simulink model "KalmanPoging1"  (R2019b)
settings: Solver=VariableStepAuto  StartTime=0.0  StopTime=6031  RelTol=1e-3
libraries: simulink x1
settings Model: Creator=pieterpinson  LastModifiedBy=pieterpinson

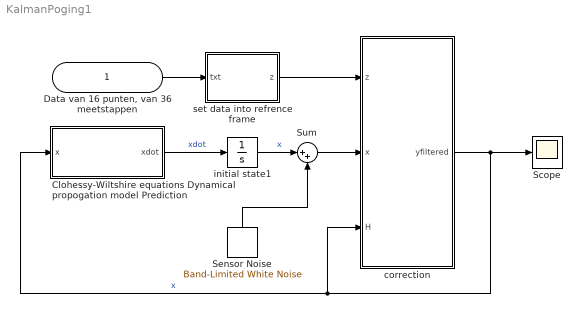
== system KalmanPoging1 ==
  "Data van 16 punten, van 36 meetstappen" : Inport
  Clohessy-Wiltshire equations Dynamical propogation model Prediction : MATLAB Function  TreatAsAtomicUnit=on
  Scope : Scope
  Sensor Noise : simulink/Sources/Band-Limited White Noise  Cov=[0.1]  Ts=0.1  seed=[23341]
  Sum : Sum  Inputs=|++
  correction : MATLAB Function  TreatAsAtomicUnit=on
  initial state1 : Integrator  InitialCondition=|
      | [-2.9671 ; 0.5236
      | ; -1.3963 ; -0.0873 ; -0.1489 ; 0.0262]
  set data into refrence frame : MATLAB Function  TreatAsAtomicUnit=on
  wires:
  "Data van 16 punten, van 36 meetstappen"/1 -> set data into refrence frame/1(txt)
  Clohessy-Wiltshire equations Dynamical propogation model Prediction/1(xdot) -> initial state1/1  "xdot"
  Sensor Noise/1 -> Sum/2
  set data into refrence frame/1(z) -> correction/1(z)
  Sum/1 -> correction/2(x)
  correction/1(yfiltered) -> Scope/1, correction/3(H), Clohessy-Wiltshire equations Dynamical propogation model Prediction/1(x)  "x"
  initial state1/1 -> Sum/1  "x"

== matlab function KalmanPoging1/set data into refrence frame ==
  data: txt input; z output
function z = measurements(txt)

    z = 239/txt;
end

== matlab function KalmanPoging1/Clohessy-Wiltshire equations Dynamical propogation model Prediction ==
  data: x input; xdot output
function xdot = SCmodel(x)

Q = 10^-6*[1 ;1 ;1];

thetadot = A*x;
omegadot = Omega*P*omega + Q;

xdot = [thetadot omegadot];

end

== matlab function KalmanPoging1/correction ==
  data: z input; x input; H input; yfiltered output
function yfiltered = Kalmanfilter(z,x,H)

    K = 0.1*[1 ; 1 ; 1];%kalman gain
    
    yfiltered = x + K*(z-H);
    
end
